simulink model "cascade_control101"  (R2024a)
settings: Solver=VariableStepAuto  StartTime=0.0  StopTime=endtime  RelTol=1e-3
undefined symbols (not defined in the file or in its folder): currentdisturbance, currentdisturbancetime, outputdisturbance, outputdisturbancetime
libraries: cstblocks x4
settings Model: Creator=barsr  LastModifiedBy=Anthony Rossiter
settings RTWCC: GPUComputeCapability=3.5

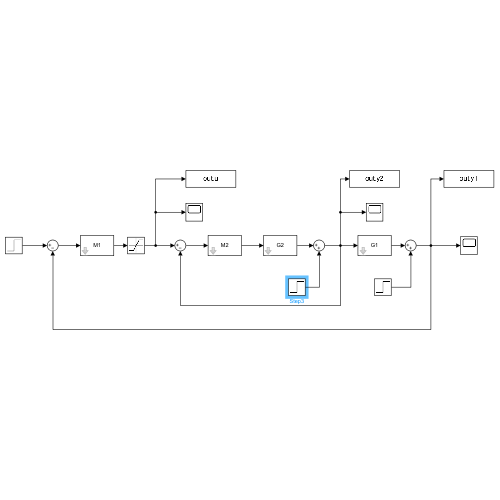
[thumbnail: Simulink's stored preview of the top-level diagram]
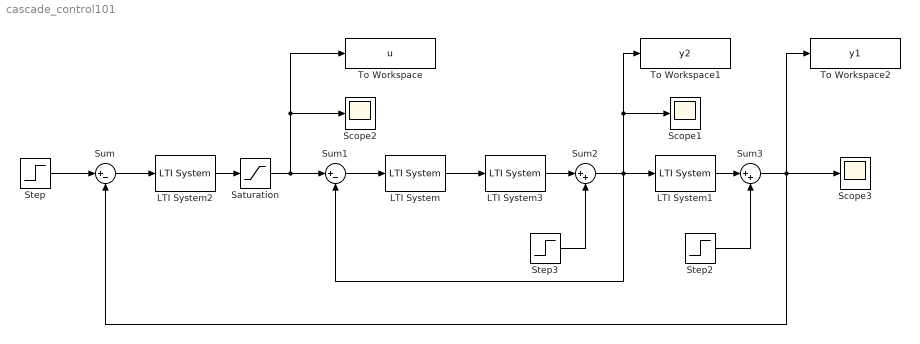
== system cascade_control101 ==
  LTI System : cstblocks/LTI System  sys=M2  IC=[]  PadeOrder=0
  LTI System1 : cstblocks/LTI System  sys=G1  IC=[]  PadeOrder=0
  LTI System2 : cstblocks/LTI System  sys=M1  IC=[]  PadeOrder=0
  LTI System3 : cstblocks/LTI System  sys=G2  IC=[]  PadeOrder=0
  Saturation : Saturate  UpperLimit=5  LowerLimit=-5
  Scope1 : Scope
  Scope2 : Scope
  Scope3 : Scope
  Step : Step  Time=0  SampleTime=0
  Step2 : Step  Time=outputdisturbancetime  After=outputdisturbance  SampleTime=0
  Step3 : Step  Time=currentdisturbancetime  After=currentdisturbance  SampleTime=0
  Sum : Sum  Inputs=|+-
  Sum1 : Sum  Inputs=|+-
  Sum2 : Sum  Inputs=|++
  Sum3 : Sum  Inputs=|++
  To Workspace : ToWorkspace  VariableName=u  SaveFormat=Structure With Time  SampleTime=-1
  To Workspace1 : ToWorkspace  VariableName=y2  SaveFormat=Structure With Time  SampleTime=-1
  To Workspace2 : ToWorkspace  VariableName=y1  SaveFormat=Structure With Time  SampleTime=-1
  wires:
  LTI System/1 -> LTI System3/1
  LTI System1/1 -> Sum3/1
  Sum/1 -> LTI System2/1
  Sum3/1 -> Scope3/1, Sum/2, To Workspace2/1
  Step3/1 -> Sum2/2
  Step2/1 -> Sum3/2
  LTI System2/1 -> Saturation/1
  Step/1 -> Sum/1
  Saturation/1 -> Scope2/1, To Workspace/1, Sum1/1
  Sum1/1 -> LTI System/1
  LTI System3/1 -> Sum2/1
  Sum2/1 -> To Workspace1/1, Scope1/1, Sum1/2, LTI System1/1
